simulink model "Algorithme_couple_precalcule"  (R2022b)
settings: Solver=VariableStepAuto  StartTime=0.0  StopTime=10.0  RelTol=1e-3
undefined symbols (not defined in the file): l1, l2, m1, m2
libraries: simulink x2
settings Model: Creator=cheye  LastModifiedBy=cheye

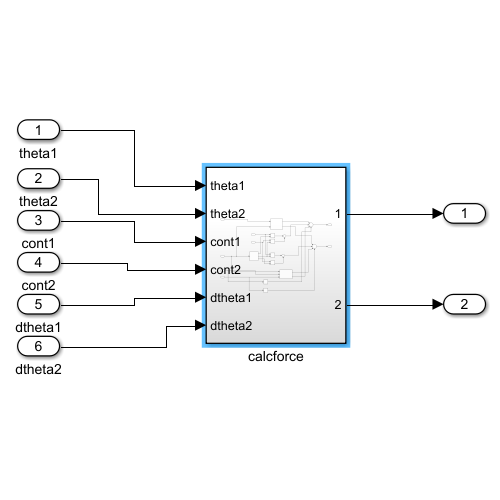
[thumbnail: Simulink's stored preview of the top-level diagram]
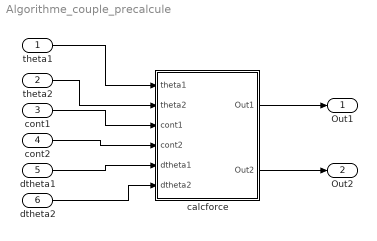
== system Algorithme_couple_precalcule ==
  theta1 : Inport
  theta2 : Inport  Port=2
  cont1 : Inport  Port=3
  cont2 : Inport  Port=4
  dtheta1 : Inport  Port=5
  dtheta2 : Inport  Port=6
  calcforce : Subsystem
  Out1 : Outport
  Out2 : Outport  Port=2
  wires:
  theta1/1 -> calcforce/1(theta1)
  theta2/1 -> calcforce/2(theta2)
  cont1/1 -> calcforce/3(cont1)
  cont2/1 -> calcforce/4(cont2)
  dtheta1/1 -> calcforce/5(dtheta1)
  dtheta2/1 -> calcforce/6(dtheta2)
  calcforce/1(Out1) -> Out1/1
  calcforce/2(Out2) -> Out2/1

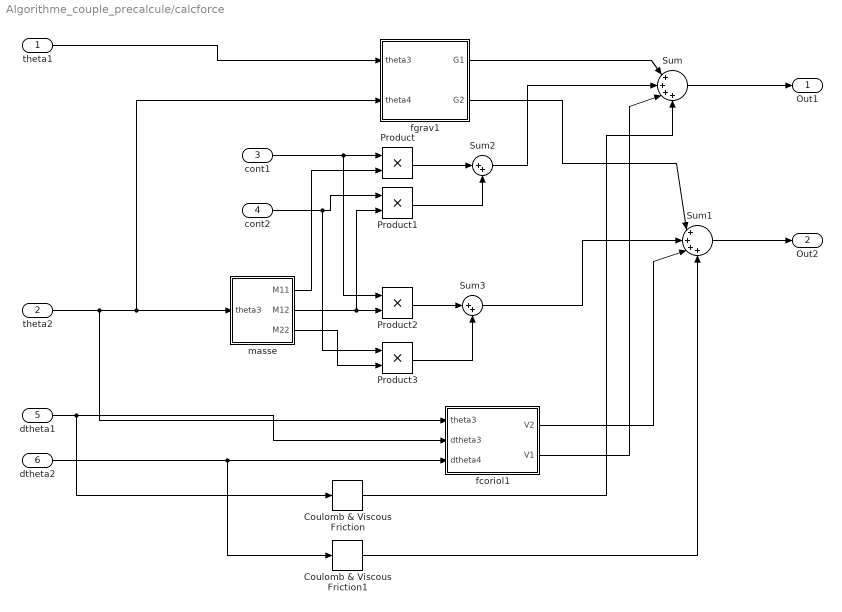
== system Algorithme_couple_precalcule/calcforce ==
  theta1 : Inport
  theta2 : Inport  Port=2
  cont1 : Inport  Port=3
  cont2 : Inport  Port=4
  dtheta1 : Inport  Port=5
  dtheta2 : Inport  Port=6
  Coulomb & Viscous Friction : simulink/Discontinuities/Coulomb & Viscous Friction  offset=[1 3 2 0]  gain=1
  Coulomb & Viscous Friction1 : simulink/Discontinuities/Coulomb & Viscous Friction  offset=[1 3 2 0]  gain=1
  Product{,1..3} (4 alike) : Product
  Sum : Sum  Inputs=|++++
  Sum1 : Sum  Inputs=|++++
  Sum2 : Sum  Inputs=|++
  Sum3 : Sum  Inputs=|++
  fcoriol1 : Subsystem
  fgrav1 : Subsystem
  masse : Subsystem
  Out1 : Outport
  Out2 : Outport  Port=2
  wires:
  fcoriol1/2(V1) -> Sum/3
  theta2/1 -> fcoriol1/1(theta3), fgrav1/2(theta4), masse/1(theta3)
  Sum2/1 -> Sum/2
  Product/1 -> Sum2/1
  Sum3/1 -> Sum1/2
  dtheta1/1 -> Coulomb & Viscous Friction/1, fcoriol1/2(dtheta3)
  cont2/1 -> Product3/1, Product1/1
  cont1/1 -> Product2/1, Product/1
  fgrav1/2(G2) -> Sum1/1
  Coulomb & Viscous Friction1/1 -> Sum1/4
  Sum1/1 -> Out2/1
  masse/3(M22) -> Product3/2
  dtheta2/1 -> Coulomb & Viscous Friction1/1, fcoriol1/3(dtheta4)
  fgrav1/1(G1) -> Sum/1
  theta1/1 -> fgrav1/1(theta3)
  masse/1(M11) -> Product/2
  Sum/1 -> Out1/1
  masse/2(M12) -> Product1/2, Product2/2
  Coulomb & Viscous Friction/1 -> Sum/4
  Product3/1 -> Sum3/2
  Product1/1 -> Sum2/2
  Product2/1 -> Sum3/1
  fcoriol1/1(V2) -> Sum1/3

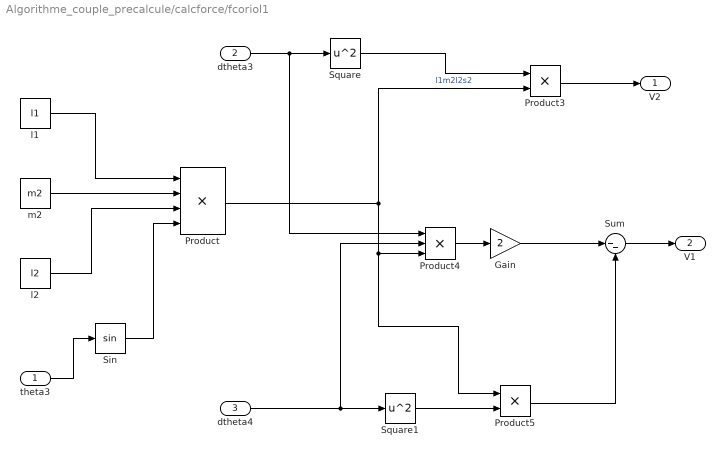
== system Algorithme_couple_precalcule/calcforce/fcoriol1 ==
  theta3 : Inport
  dtheta3 : Inport  Port=2
  dtheta4 : Inport  Port=3
  Gain : Gain  Gain=2
  Product : Product  Inputs=4
  Product3 : Product
  Product4 : Product  Inputs=3
  Product5 : Product
  Sin : Trigonometry
  Square : Math  Operator=square
  Square1 : Math  Operator=square
  Sum : Sum  Inputs=|--
  l1 : Constant  Value=l1
  l2 : Constant  Value=l2
  m2 : Constant  Value=m2
  V2 : Outport
  V1 : Outport  Port=2
  wires:
  Gain/1 -> Sum/1
  m2/1 -> Product/2
  l1/1 -> Product/1
  theta3/1 -> Sin/1
  dtheta4/1 -> Square1/1, Product4/2
  dtheta3/1 -> Product4/1, Square/1
  l2/1 -> Product/3
  Sum/1 -> V1/1
  Product4/1 -> Gain/1
  Product5/1 -> Sum/2
  Square/1 -> Product3/1
  Product/1 -> Product4/3, Product5/1, Product3/2  "l1m2l2s2"
  Product3/1 -> V2/1
  Sin/1 -> Product/4
  Square1/1 -> Product5/2

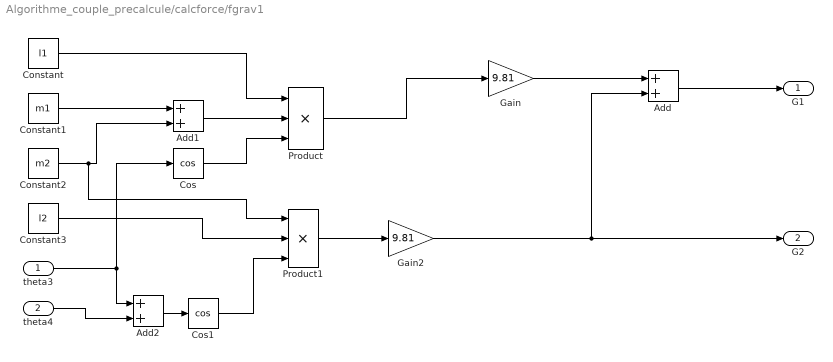
== system Algorithme_couple_precalcule/calcforce/fgrav1 ==
  theta3 : Inport
  theta4 : Inport  Port=2
  Add : Sum
  Add1 : Sum
  Add2 : Sum
  Constant : Constant  Value=l1
  Constant1 : Constant  Value=m1
  Constant2 : Constant  Value=m2
  Constant3 : Constant  Value=l2
  Cos : Trigonometry  Operator=cos
  Cos1 : Trigonometry  Operator=cos
  Gain : Gain  Gain=9.81
  Gain2 : Gain  Gain=9.81
  Product : Product  Inputs=3
  Product1 : Product  Inputs=3
  G1 : Outport
  G2 : Outport  Port=2
  wires:
  Add/1 -> G1/1
  Constant1/1 -> Add1/1
  Add2/1 -> Cos1/1
  Product/1 -> Gain/1
  Cos1/1 -> Product1/3
  Constant/1 -> Product/1
  Add1/1 -> Product/2
  Gain/1 -> Add/1
  Constant2/1 -> Product1/1, Add1/2
  Cos/1 -> Product/3
  theta4/1 -> Add2/2
  Gain2/1 -> G2/1, Add/2
  theta3/1 -> Cos/1, Add2/1
  Constant3/1 -> Product1/2
  Product1/1 -> Gain2/1

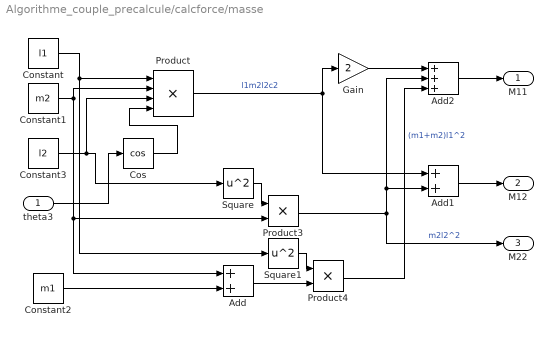
== system Algorithme_couple_precalcule/calcforce/masse ==
  theta3 : Inport
  Add : Sum
  Add1 : Sum
  Add2 : Sum  Inputs=+++
  Constant : Constant  Value=l1
  Constant1 : Constant  Value=m2
  Constant2 : Constant  Value=m1
  Constant3 : Constant  Value=l2
  Cos : Trigonometry  Operator=cos
  Gain : Gain  Gain=2
  Product : Product  Inputs=4
  Product3 : Product
  Product4 : Product
  Square : Math  Operator=square
  Square1 : Math  Operator=square
  M11 : Outport
  M12 : Outport  Port=2
  M22 : Outport  Port=3
  wires:
  Constant/1 -> Product/1, Square1/1
  Add2/1 -> M11/1
  Product/1 -> Add1/1, Gain/1  "l1m2l2c2"
  Constant1/1 -> Product/2, Add/1, Product3/2
  Constant3/1 -> Product/3, Square/1
  Cos/1 -> Product/4
  Product3/1 -> M22/1, Add2/2, Add1/2  "m2l2^2"
  Add/1 -> Product4/2
  Product4/1 -> Add2/3  "(m1+m2)l1^2"
  Constant2/1 -> Add/2
  Gain/1 -> Add2/1
  Square1/1 -> Product4/1
  Square/1 -> Product3/1
  theta3/1 -> Cos/1
  Add1/1 -> M12/1
